simulink model "Modelo2R2021a"  (R2021a)
settings: Solver=VariableStepAuto  StartTime=0.0  StopTime=7e4  FixedStep=1  MaxStep=1  RelTol=1e-3
PostLoadFcn:
  | load('input_modelo_bateria.mat')
undefined symbols (not defined in the file or in its folder): alfa, beta, Cn, rest_time, SOC_MAX, SOC_MIN, Temperature, voc_fit
libraries: fl_lib x8, nesl_utility x7, ee_lib x2, simulink x1
settings Model: PacingRate=1000  Creator=eduardo.guimaraes  LastModifiedBy=mateu
settings SolverCC: AlgebraicLoopSolver=TrustRegion
settings DataIOCC: ReturnWorkspaceOutputs=off
settings DebuggingCC: SFMachineParentedDataDiag=warning  ArithmeticOperatorsInVariantConditions=warning
settings SFSimCC: CustomCodeUndefinedFunction=UseInterfaceOnly

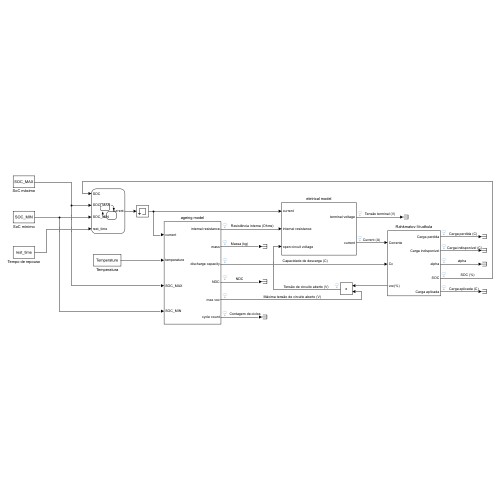
[thumbnail: Simulink's stored preview of the top-level diagram]
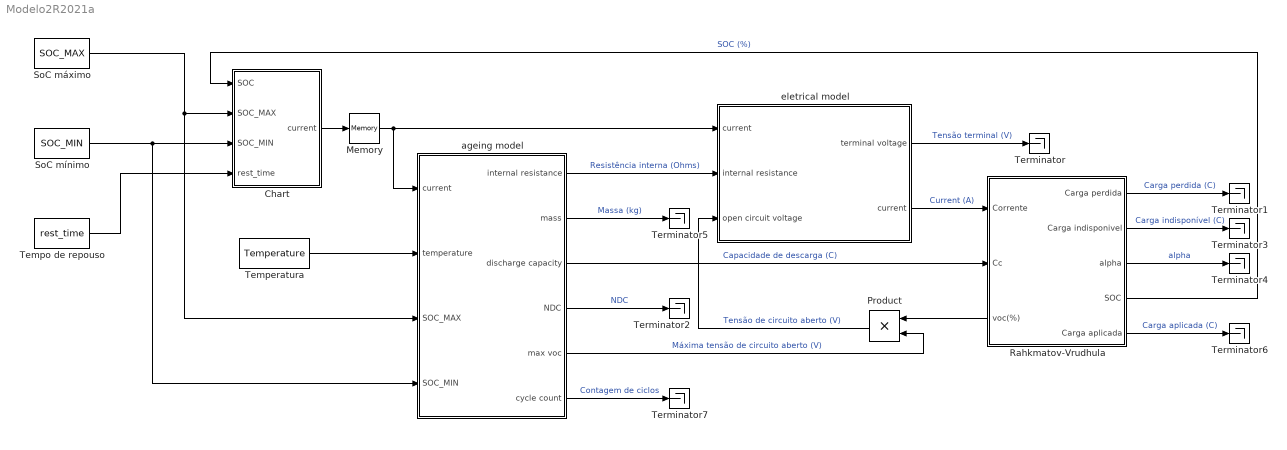
== system Modelo2R2021a ==
  Chart : Stateflow chart  TreatAsAtomicUnit=on
      settings: PortSchema="{\"entries\":[{\"content\":{\"sides\":[{\"content\":{\"connectorIds\":[\"In2\",\"In3\",\"In4\",\"In1\"]},\"type\":\"ConnectorPlacement.EquallySpacedRectSide\",\"uuid\":\"b79e6304-446b-4da0-b841-6a7e0125cfd5\"},{\"content\":{\"connectorIds\":[\"Out1\"],\"side\":\"RIGHT\"},\"type\":\"ConnectorPlacement.EquallySpacedRectSide\",\"uuid\":\"907ab61a-1d0a-45c7-8983-f54ad408e9d5\"},{\"content\":{\"connectorIds\":[],\"side\":\"TOP\"},\"type\":\"ConnectorPlacement.EquallySpacedRectSide\",\"uuid\":\"544cfd83-6b45-4625-b149-12de8a160085\"}]},\"type\":\"ConnectorPlacement.EquallySpacedConnector\",\"uuid\":\"2fa71fdc-98f6-47db-8b29-348eadeade42\"}],\"packageUris\":[\"http://schema.mathworks.com/mf0/Connector/R2020b\"],\"version\":\"1.0\"}"
  Memory : Memory
  Product : Product
  Rahkmatov-Vrudhula : Subsystem
      settings: PortSchema="{\"entries\":[{\"content\":{\"sides\":[{\"content\":{\"connectorIds\":[\"In1\",\"In2\",\"Out6\"]},\"type\":\"ConnectorPlacement.EquallySpacedRectSide\",\"uuid\":\"83f3e873-db9f-47d1-b7c3-7eda48a10b32\"},{\"content\":{\"connectorIds\":[\"Out1\",\"Out2\",\"Out3\",\"Out4\",\"Out5\"],\"side\":\"RIGHT\"},\"type\":\"ConnectorPlacement.EquallySpacedRectSide\",\"uuid\":\"48ac6012-cdb4-4752-bc48-afa50bea9f0a\"},{\"content\":{\"connectorIds\":[],\"side\":\"TOP\"},\"type\":\"ConnectorPlacement.EquallySpacedRectSide\",\"uuid\":\"9cdc78bf-a718-48f1-92e6-e4070151caee\"}]},\"type\":\"ConnectorPlacement.EquallySpacedConnector\",\"uuid\":\"a231f58d-8e16-4cb4-bc80-61541bcf90eb\"}],\"packageUris\":[\"http://schema.mathworks.com/mf0/Connector/R2020b\"],\"version\":\"1.0\"}"
  SoC máximo : Constant  Value=SOC_MAX
  SoC mínimo : Constant  Value=SOC_MIN
  Temperatura : Constant  Value=Temperature
  Tempo de repouso : Constant  Value=rest_time
  Terminator{,1..7} (8 alike) : Terminator
  ageing model : Subsystem
  eletrical model : Subsystem
  wires:
  Temperatura/1 -> ageing model/2(temperature)
  Rahkmatov-Vrudhula/4(SOC) -> Chart/2(SOC)  "SOC (%)"
  Tempo de repouso/1 -> Chart/1(rest_time)
  ageing model/3(discharge capacity) -> Rahkmatov-Vrudhula/2(Cc)  "Capacidade de descarga (C)"
  Chart/1(current) -> Memory/1
  Memory/1 -> eletrical model/1("current "), ageing model/1(current)
  SoC máximo/1 -> ageing model/3(SOC_MAX), Chart/3(SOC_MAX)
  SoC mínimo/1 -> ageing model/4(SOC_MIN), Chart/4(SOC_MIN)
  eletrical model/2(current) -> Rahkmatov-Vrudhula/1(Corrente)  "Current (A)"
  ageing model/1(internal resistance) -> eletrical model/2(internal resistance)  "Resistência interna (Ohms)"
  Rahkmatov-Vrudhula/6(voc(%)) -> Product/1
  ageing model/5(max voc) -> Product/2  "Máxima tensão de circuito aberto (V)"
  Product/1 -> eletrical model/3(open circuit voltage)  "Tensão de circuito aberto (V)"
  eletrical model/1(terminal voltage) -> Terminator/1  "Tensão terminal (V)"
  Rahkmatov-Vrudhula/1(Carga perdida) -> Terminator1/1  "Carga perdida (C)"
  Rahkmatov-Vrudhula/2(Carga indisponivel) -> Terminator3/1  "Carga indisponível (C)"
  Rahkmatov-Vrudhula/3(alpha) -> Terminator4/1  "alpha"
  ageing model/4(NDC) -> Terminator2/1  "NDC"
  ageing model/2(mass) -> Terminator5/1  "Massa (kg)"
  Rahkmatov-Vrudhula/5(Carga aplicada) -> Terminator6/1  "Carga aplicada (C)"
  ageing model/6(cycle count) -> Terminator7/1  "Contagem de ciclos"

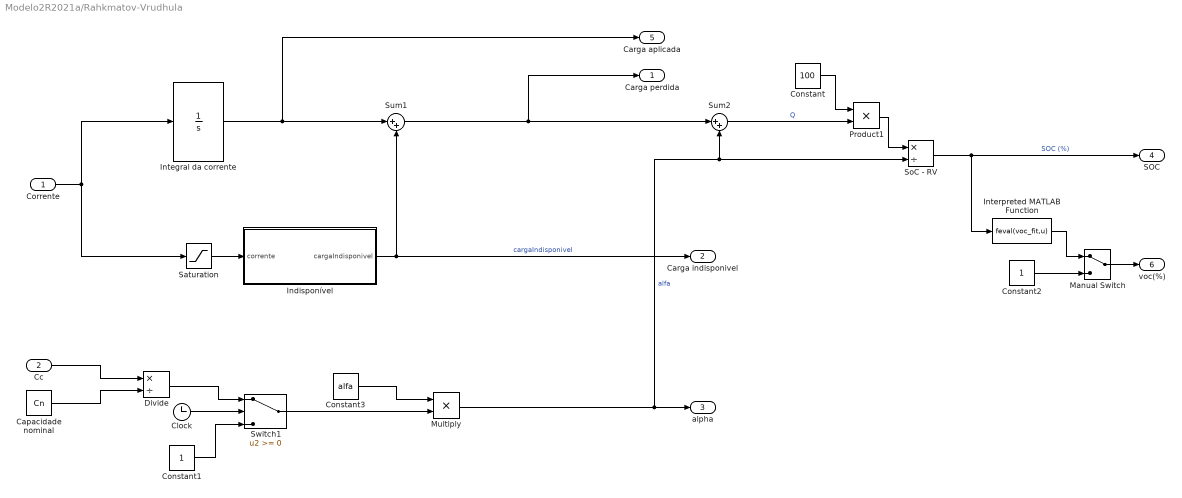
== system Modelo2R2021a/Rahkmatov-Vrudhula ==
  Corrente : Inport
  Cc : Inport  Port=2
  Capacidade nominal : Constant  Value=Cn
  Clock : Clock
  Constant : Constant  Value=100
  Constant1 : Constant
  Constant2 : Constant
  Constant3 : Constant  Value=alfa
  Divide : Product  Inputs=*/
  Indisponível : Subsystem
  Integral da corrente : Integrator  LimitOutput=on  UpperSaturationLimit=0  LowerSaturationLimit=-alfa
  Interpreted MATLAB Function : MATLABFcn  MATLABFcn=feval(voc_fit,u)
  Manual Switch : ManualSwitch
  Multiply : Product
  Product1 : Product
  Saturation : Saturate  UpperLimit=0  LowerLimit=-Inf
  SoC - RV : Product  Inputs=*/
  Sum1 : Sum  Inputs=|++
  Sum2 : Sum  Inputs=|++
  Switch1 : Switch
  Carga perdida : Outport  VectorParamsAs1DForOutWhenUnconnected=off
  Carga indisponivel : Outport  Port=2  VectorParamsAs1DForOutWhenUnconnected=off
  alpha : Outport  Port=3  VectorParamsAs1DForOutWhenUnconnected=off
  SOC : Outport  Port=4
  Carga aplicada : Outport  Port=5  VectorParamsAs1DForOutWhenUnconnected=off
  voc(%) : Outport  Port=6
  wires:
  Indisponível/1(cargaIndisponivel) -> Sum1/2, Carga indisponivel/1  "cargaIndisponivel"
  Switch1/1 -> Multiply/2
  Constant3/1 -> Multiply/1
  Constant/1 -> Product1/1
  Multiply/1 -> Sum2/2, SoC - RV/2, alpha/1  "alfa"
  Product1/1 -> SoC - RV/1
  SoC - RV/1 -> Interpreted MATLAB Function/1, SOC/1  "SOC (%)"
  Saturation/1 -> Indisponível/1(corrente)
  Sum2/1 -> Product1/2  "Q"
  Constant1/1 -> Switch1/3
  Clock/1 -> Switch1/2
  Divide/1 -> Switch1/1
  Cc/1 -> Divide/1
  Capacidade nominal/1 -> Divide/2
  Integral da corrente/1 -> Carga aplicada/1, Sum1/1
  Corrente/1 -> Integral da corrente/1, Saturation/1
  Sum1/1 -> Carga perdida/1, Sum2/1
  Manual Switch/1 -> voc(%)/1
  Interpreted MATLAB Function/1 -> Manual Switch/1
  Constant2/1 -> Manual Switch/2

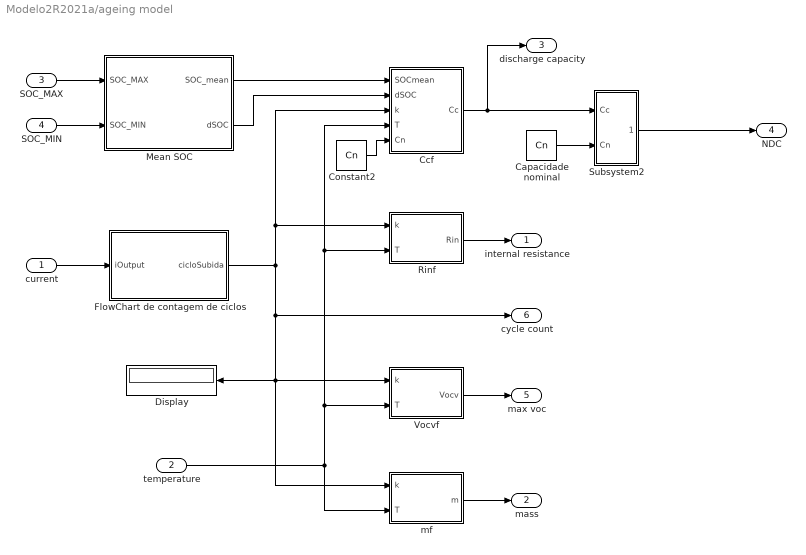
== system Modelo2R2021a/ageing model ==
  current : Inport
  temperature : Inport  Port=2
  SOC_MAX : Inport  Port=3
  SOC_MIN : Inport  Port=4
  Capacidade nominal : Constant  Value=Cn
  Ccf : MATLAB Function  TreatAsAtomicUnit=on
  Constant2 : Constant  Value=Cn
  Display : Display
  FlowChart de contagem de ciclos : Stateflow chart  TreatAsAtomicUnit=on
  Mean SOC : Subsystem
  Rinf : MATLAB Function  TreatAsAtomicUnit=on
  Subsystem2 : Subsystem
  Vocvf : MATLAB Function  TreatAsAtomicUnit=on
  mf : MATLAB Function  TreatAsAtomicUnit=on
  internal resistance : Outport
  mass : Outport  Port=2
  discharge capacity : Outport  Port=3
  NDC : Outport  Port=4
  max voc : Outport  Port=5
  cycle count : Outport  Port=6
  wires:
  Vocvf/1(Vocv) -> max voc/1
  temperature/1 -> mf/2(T), Vocvf/2(T), Rinf/2(T), Ccf/4(T)
  Rinf/1(Rin) -> internal resistance/1
  mf/1(m) -> mass/1
  current/1 -> FlowChart de contagem de ciclos/1(iOutput)
  Ccf/1(Cc) -> discharge capacity/1, Subsystem2/1(Cc)
  Subsystem2/1(NDC) -> NDC/1
  Capacidade nominal/1 -> Subsystem2/2(Cn)
  Constant2/1 -> Ccf/5(Cn)
  SOC_MAX/1 -> Mean SOC/1(SOC_MAX)
  SOC_MIN/1 -> Mean SOC/2(SOC_MIN)
  Mean SOC/1(SOC_mean) -> Ccf/1(SOCmean)
  Mean SOC/2(dSOC) -> Ccf/2(dSOC)
  FlowChart de contagem de ciclos/1(cicloSubida) -> Ccf/3(k), Rinf/1(k), cycle count/1, Display/1, mf/1(k), Vocvf/1(k)

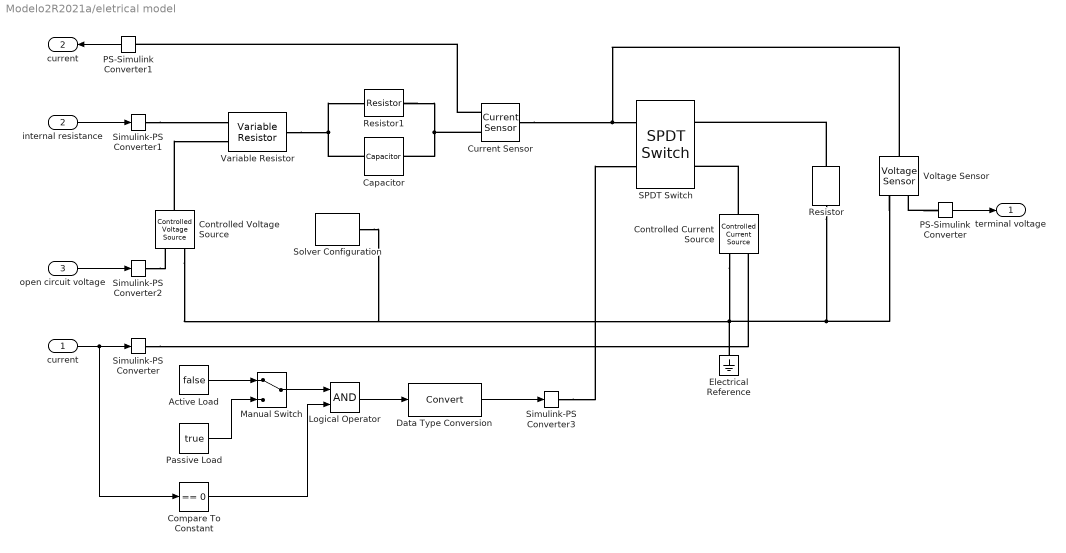
== system Modelo2R2021a/eletrical model ==
  "current " : Inport
  internal resistance : Inport  Port=2
  open circuit voltage : Inport  Port=3
  Active Load : Constant  Value=false
  Capacitor : fl_lib/Electrical/Electrical Elements/Capacitor  c=500 F  r=1e-6 Ohm  g=0 1/Ohm  i_specify=off  i_priority=None  i=0 A  i_nominal_specify=off  i_nominal_unit=A  i_nominal_value=1  v_specify=off  v_priority=None  v=0 V  v_nominal_specify=off  v_nominal_unit=V  v_nominal_value=1  vc_specify=off  vc_priority=High  vc=0 V  vc_nominal_specify=off  vc_nominal_unit=V  vc_nominal_value=1
      settings: SourceProductBaseCode=PW,SS,VE
  Compare To Constant : simulink/Logic and Bit Operations/Compare To Constant  relop===  const=0  OutDataTypeStr=boolean
  Controlled Current Source : fl_lib/Electrical/Electrical Sources/Controlled Current Source
      settings: SourceProductBaseCode=PW,SS,VE
  Controlled Voltage Source : fl_lib/Electrical/Electrical Sources/Controlled Voltage Source
      settings: SourceProductBaseCode=PW,SS,VE
  Current Sensor : fl_lib/Electrical/Electrical Sensors/Current Sensor
      settings: SourceProductBaseCode=PW,SS,VE
  Data Type Conversion : DataTypeConversion
  Electrical Reference : fl_lib/Electrical/Electrical Elements/Electrical Reference
      settings: SourceProductBaseCode=PW,SS,VE
  Logical Operator : Logic  AllPortsSameDT=off  OutDataTypeStr=boolean
  Manual Switch : ManualSwitch
  PS-Simulink Converter : nesl_utility/PS-Simulink Converter  PhysicalDomain=network_engine_domain  SubClassName=ps_output  LeftPortType=input  RightPortType=output  PseudoPeriodic=off  Frequencies=[]  VectorFormat=inherit  Unit=inherit  AffineConversion=off
      settings: SourceProductBaseCode=SS,PW,VE
  PS-Simulink Converter1 : nesl_utility/PS-Simulink Converter  PhysicalDomain=network_engine_domain  SubClassName=ps_output  LeftPortType=input  RightPortType=output  PseudoPeriodic=off  Frequencies=[]  VectorFormat=inherit  Unit=inherit  AffineConversion=off
      settings: SourceProductBaseCode=SS,PW,VE
  Passive Load : Constant  Value=true
  Resistor : ee_lib/Passive/Resistor  R=0.1 Ohm  enable_R_tol=0  R_tol=5  tol_distribution=1  nSigma=4  enable_operating_limits=0  operating_limit_action=2  max_working_voltage=100 V  power_rating=1 W  enable_faults=0  fault_action=1  R_faulted=inf Ohm  enable_temporal_fault=0  t_fault=1 s  enable_behavioral_fault=0  max_permissible_current=1 A  t_fail_on_current=1 s  noise_mode=0  sample_time=1e-3 s  repeatability=1  auto_seed=3499211588  user_seed=0  Tdevice=25 degC  power_derating_T1=70 degC  power_derating_T2=155 degC  operating_temperature_range_vec=[-50, 150] degC  alpha=3.93e-3 1/K  Tmeas=25 degC  thermal_mass=100 J/K  temperature_specify=off  temperature_priority=High  temperature=298.15 K  temperature_nominal_specify=off  temperature_nominal_unit=K  temperature_nominal_value=1
  Resistor1 : fl_lib/Electrical/Electrical Elements/Resistor  R=1e-6 Ohm  i_specify=off  i_priority=None  i=0 A  i_nominal_specify=off  i_nominal_unit=A  i_nominal_value=1  v_specify=off  v_priority=None  v=0 V  v_nominal_specify=off  v_nominal_unit=V  v_nominal_value=1
      settings: SourceProductBaseCode=PW,SS,VE
  SPDT Switch : ee_lib/Switches & Breakers/SPDT Switch  R_closed=0.01 Ohm  G_open=1e-6 S  Threshold=0.5 V  Width=0 V  model_dynamics=0  t_on=1e-3 s  t_off=1e-3 s  initial_vT=0 V
      settings: SourceProductBaseCode=PS
  Simulink-PS Converter : nesl_utility/Simulink-PS Converter  PhysicalDomain=network_engine_domain  SubClassName=ps_input  LeftPortType=input  RightPortType=output  PseudoPeriodic=off  Frequencies=[]  NoiseDistribution=none  NoiseParameters=[]  Unit=1  AffineConversion=off  FilteringAndDerivatives=zero  SimscapeFilterOrder=1  InputFilterTimeConstant=0.001  UdotUserProvided=0
      settings: SourceProductBaseCode=SS,PW,VE
  Simulink-PS Converter1 : nesl_utility/Simulink-PS Converter  PhysicalDomain=network_engine_domain  SubClassName=ps_input  LeftPortType=input  RightPortType=output  PseudoPeriodic=off  Frequencies=[]  NoiseDistribution=none  NoiseParameters=[]  Unit=1  AffineConversion=off  FilteringAndDerivatives=zero  SimscapeFilterOrder=1  InputFilterTimeConstant=0.001  UdotUserProvided=0
      settings: SourceProductBaseCode=SS,PW,VE
  Simulink-PS Converter2 : nesl_utility/Simulink-PS Converter  PhysicalDomain=network_engine_domain  SubClassName=ps_input  LeftPortType=input  RightPortType=output  PseudoPeriodic=off  Frequencies=[]  NoiseDistribution=none  NoiseParameters=[]  Unit=1  AffineConversion=off  FilteringAndDerivatives=zero  SimscapeFilterOrder=1  InputFilterTimeConstant=0.001  UdotUserProvided=0
      settings: SourceProductBaseCode=SS,PW,VE
  Simulink-PS Converter3 : nesl_utility/Simulink-PS Converter  PhysicalDomain=network_engine_domain  SubClassName=ps_input  LeftPortType=input  RightPortType=output  PseudoPeriodic=off  Frequencies=[]  NoiseDistribution=none  NoiseParameters=[]  Unit=1  AffineConversion=off  FilteringAndDerivatives=provide  SimscapeFilterOrder=1  InputFilterTimeConstant=0.001  UdotUserProvided=0
      settings: SourceProductBaseCode=SS,PW,VE
  Solver Configuration : nesl_utility/Solver Configuration  PhysicalDomain=network_engine_domain  SubClassName=solver  LeftPortType=input  RightPortType=generic  Tones=[]  Harmonics=[]  SimulateNoise=off  Profile=off  UseLocalSampling=off  EnableSwitchedLinearOptims=on  FrequencyDomain=off  UseCCode=off  RelTol=0.001  AbsTol=0.001  MinStep=1e-09  ToWorkspace=off  RevertToSquareIcSolve=off  NumHomotopyIterations=100  PhasorMode=off  PhasorModeNumHarmonics=1  IndexReductionMethod=DerivativeReplacement  DoDC=off  ResidualTolerance=1e-09  UseLocalSolver=off  LocalSolverChoice=NE_BACKWARD_EULER_ADVANCER  LocalSolverSampleTime=0.001  DoFixedCost=off  MaxNonlinIter=3  MaxModeIter=2  ComputeImpulses=off  ImpulseIterations=2  LinearAlgebra=auto  LinearAlgebraNumThread=0  EquationFormulation=NE_TIME_EF  DelaysMemoryBudget=1024  AutomaticFiltering=on  FilteringTimeConstant=0.001  PartitionStorageMethod=AS_NEEDED  PartitionMemoryBudget=1024  PartitionMethod=ROBUST
      settings: SourceProductBaseCode=SS,PW,VE
  Variable Resistor : fl_lib/Electrical/Electrical Elements/Variable Resistor  Rmin=0 Ohm  i_specify=off  i_priority=None  i=0 A  i_nominal_specify=off  i_nominal_unit=A  i_nominal_value=1  v_specify=off  v_priority=None  v=0 V  v_nominal_specify=off  v_nominal_unit=V  v_nominal_value=1
      settings: SourceProductBaseCode=PW,SS,VE
  Voltage Sensor : fl_lib/Electrical/Electrical Sensors/Voltage Sensor
      settings: SourceProductBaseCode=PW,SS,VE
  terminal voltage : Outport
  current : Outport  Port=2
  wires:
  open circuit voltage/1 -> Simulink-PS Converter2/1
  "current "/1 -> Compare To Constant/1, Simulink-PS Converter/1
  PS-Simulink Converter1/1 -> current/1
  internal resistance/1 -> Simulink-PS Converter1/1
  PS-Simulink Converter/1 -> terminal voltage/1
  Compare To Constant/1 -> Logical Operator/2
  Logical Operator/1 -> Data Type Conversion/1
  Data Type Conversion/1 -> Simulink-PS Converter3/1
  Active Load/1 -> Manual Switch/1
  Passive Load/1 -> Manual Switch/2
  Manual Switch/1 -> Logical Operator/1
  connections:
  Variable Resistor/RConn1 -- Capacitor/LConn1 -- Resistor1/LConn1
  Voltage Sensor/RConn2 -- Controlled Voltage Source/RConn2 -- Solver Configuration/RConn1 -- Controlled Current Source/RConn2 -- Electrical Reference/LConn1 -- Resistor/RConn1
  Controlled Voltage Source/LConn1 -- Variable Resistor/LConn2
  Simulink-PS Converter/RConn1 -- Controlled Current Source/RConn1
  PS-Simulink Converter/LConn1 -- Voltage Sensor/RConn1
  Simulink-PS Converter1/RConn1 -- Variable Resistor/LConn1
  Simulink-PS Converter2/RConn1 -- Controlled Voltage Source/RConn1
  Resistor1/RConn1 -- Current Sensor/RConn2 -- Capacitor/RConn1
  Voltage Sensor/LConn1 -- Current Sensor/LConn1 -- SPDT Switch/LConn2
  Current Sensor/RConn1 -- PS-Simulink Converter1/LConn1
  Controlled Current Source/LConn1 -- SPDT Switch/RConn1
  Resistor/LConn1 -- SPDT Switch/RConn2
  Simulink-PS Converter3/RConn1 -- SPDT Switch/LConn1

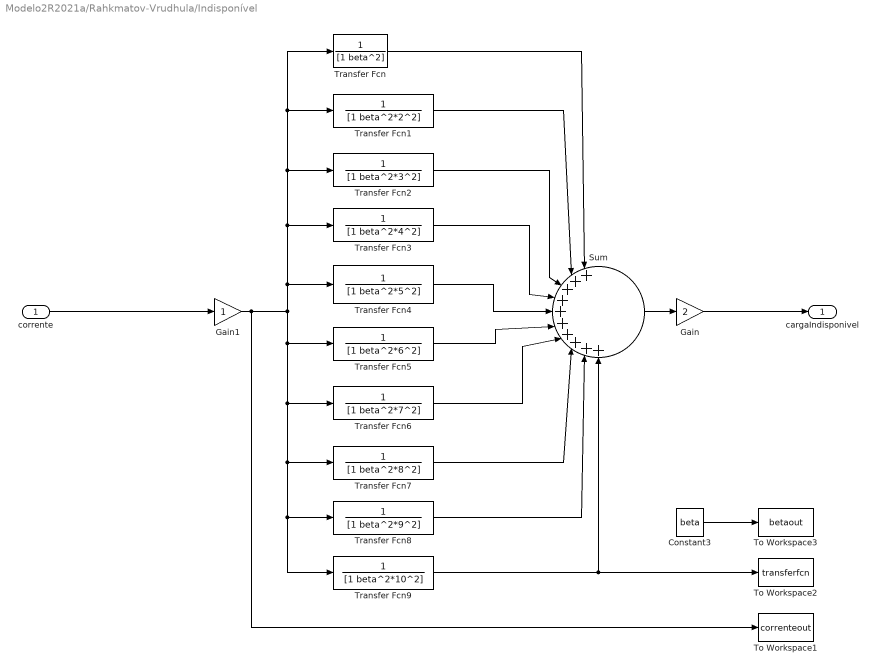
== system Modelo2R2021a/Rahkmatov-Vrudhula/Indisponível ==
  corrente : Inport
  Constant3 : Constant  Value=beta
  Gain : Gain  Gain=2
  Gain1 : Gain
  Sum : Sum  Inputs=|++++++++++
  To Workspace1 : ToWorkspace  VariableName=correnteout  SampleTime=-1
      settings: Save2DSignal=2-D array (concatenate along first dimension)
  To Workspace2 : ToWorkspace  VariableName=transferfcn  SampleTime=-1
      settings: Save2DSignal=2-D array (concatenate along first dimension)
  To Workspace3 : ToWorkspace  VariableName=betaout  SampleTime=-1
      settings: Save2DSignal=2-D array (concatenate along first dimension)
  Transfer Fcn : TransferFcn  Denominator=[1 beta^2]
  Transfer Fcn1 : TransferFcn  Denominator=[1 beta^2*2^2]
  Transfer Fcn2 : TransferFcn  Denominator=[1 beta^2*3^2]
  Transfer Fcn3 : TransferFcn  Denominator=[1 beta^2*4^2]
  Transfer Fcn4 : TransferFcn  Denominator=[1 beta^2*5^2]
  Transfer Fcn5 : TransferFcn  Denominator=[1 beta^2*6^2]
  Transfer Fcn6 : TransferFcn  Denominator=[1 beta^2*7^2]
  Transfer Fcn7 : TransferFcn  Denominator=[1 beta^2*8^2]
  Transfer Fcn8 : TransferFcn  Denominator=[1 beta^2*9^2]
  Transfer Fcn9 : TransferFcn  Denominator=[1 beta^2*10^2]
  cargaIndisponivel : Outport  VectorParamsAs1DForOutWhenUnconnected=off
  wires:
  Transfer Fcn/1 -> Sum/1
  Transfer Fcn1/1 -> Sum/2
  Transfer Fcn2/1 -> Sum/3
  Transfer Fcn3/1 -> Sum/4
  Transfer Fcn4/1 -> Sum/5
  Transfer Fcn5/1 -> Sum/6
  Transfer Fcn6/1 -> Sum/7
  Transfer Fcn7/1 -> Sum/8
  Transfer Fcn8/1 -> Sum/9
  Transfer Fcn9/1 -> To Workspace2/1, Sum/10
  Sum/1 -> Gain/1
  Gain1/1 -> To Workspace1/1, Transfer Fcn5/1, Transfer Fcn6/1, Transfer Fcn7/1, Transfer Fcn8/1, Transfer Fcn9/1, Transfer Fcn4/1, Transfer Fcn3/1, Transfer Fcn2/1, Transfer Fcn1/1, Transfer Fcn/1
  corrente/1 -> Gain1/1
  Gain/1 -> cargaIndisponivel/1
  Constant3/1 -> To Workspace3/1

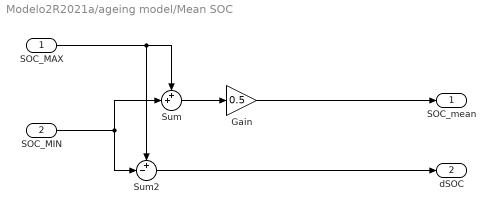
== system Modelo2R2021a/ageing model/Mean SOC ==
  SOC_MAX : Inport
  SOC_MIN : Inport  Port=2
  Gain : Gain  Gain=0.5
  Sum : Sum  Inputs=++|
  Sum2 : Sum  Inputs=+-|
  SOC_mean : Outport
  dSOC : Outport  Port=2
  wires:
  Sum/1 -> Gain/1
  SOC_MIN/1 -> Sum/2, Sum2/2
  SOC_MAX/1 -> Sum/1, Sum2/1
  Sum2/1 -> dSOC/1
  Gain/1 -> SOC_mean/1

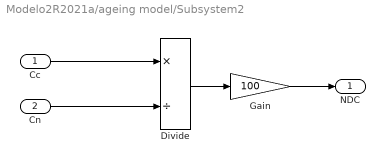
== system Modelo2R2021a/ageing model/Subsystem2 ==
  Cc : Inport
  Cn : Inport  Port=2
  Divide : Product  Inputs=*/
  Gain : Gain  Gain=100
  NDC : Outport
  wires:
  Divide/1 -> Gain/1
  Cn/1 -> Divide/2
  Gain/1 -> NDC/1
  Cc/1 -> Divide/1

== matlab function Modelo2R2021a/ageing model/Rinf ==
  data: k input; Rin output; T input
function Rin = fcn(k,T)

       x = (k-9000)/6326;
       y = (T-31.67)/10.57;
       
%        where x is normalized by mean 9000 and std 6326
%        and where y is normalized by mean 31.67 and std 10.57
% Coefficients (with 95% confidence bounds):
       p00 =    0.003956;%  (0.003728, 0.004184)
       p10 =   0.0006753;%  (0.0004339, 0.0009166)
       p01 =  -1.804e-05;%  (-0.0001419, 0.0001059)
       p20 =   0.0005921;%  (0.000144, 0.00104)
       p11 =   0.0002673;%  (4.651e-05, 0.0004881)
       p02 =   3.119e-05;%  (-0.0001491, 0.0002115)
       p30 =   0.0001137;%  (-7.891e-06, 0.0002354)
       p21 =   0.0002022;%  (0.0001025, 0.0003019)
       p12 =  -0.0002286;%  (-0.0003492, -0.0001081)
       p40 =  -1.788e-05;%  (-0.0002076, 0.0001718)
       p31 =  -1.552e-05;%  (-0.0001407, 0.0001096)
       p22 =  -0.0001674;%  (-0.0003125, -2.232e-05)

       %Linear model Poly42:
     Rin = p00 + p10*x + p01*y + p20*x^2 + p11*x*y + p02*y^2 + p30*x^3 + p21*x^2*y ...
                    + p12*x*y^2 + p40*x^4 + p31*x^3*y + p22*x^2*y^2;

       
% Goodness of fit:
%   SSE: 9.784e-08
%   R-square: 0.991
%   Adjusted R-square: 0.9746
%   RMSE: 0.0001277

== matlab function Modelo2R2021a/ageing model/Ccf ==
  data: SOCmean input; dSOC input; k input; Cc output; T input; Cn input
function Cc = fcn(SOCmean, dSOC,k,T,Cn)
% Coeficients model Saxena2016
        k1 = 3.25;
        k2 = 3.25;
        k3 = -2.25;
% Coefficients (with 95% confidence bounds):
       p00 =       56.02;%  (53.93, 58.1)
       p10 =      -10.53;%  (-13.71, -7.36)
       p01 =       0.869;%  (-0.7052, 2.443)
       p20 =      -4.808;%  (-6.007, -3.609)
       p11 =      -1.445;%  (-2.534, -0.3554)
       p02 =      -1.223;%  (-2.763, 0.3179)
       p30 =      -2.931;%  (-4.53, -1.332)
       p21 =       -1.55;%  (-2.783, -0.3163)
       p12 =    -0.09181;%  (-1.677, 1.493)

       x = (k-9000)/6326;
       y = (T-31.67)/10.57;
       
%Linear model Poly32:
     fcn = p00 + p10*x + p01*y + p20*x^2 + p11*x*y + p02*y^2 + p30*x^3 + p21*x^2*y + p12*x*y^2;

     Cc = (100 - k1*SOCmean/100*(1+k2*dSOC/100+k3*(dSOC/100)^2) )/100*fcn
                    
%       where x is normalized by mean 9000 and std 6326
%       and where y is normalized by mean 31.67 and std 10.57


% Goodness of fit:
%   SSE: 29.68
%   R-square: 0.9934
%   Adjusted R-square: 0.9875
%   RMSE: 1.816

== stateflow chart Modelo2R2021a/ageing model/FlowChart de contagem de ciclos ==
  note: Automato de contagem de ciclos
  state Respouso
  state Descarregando
  state Carregando
  (default) -> Respouso
  Respouso -> Descarregando [order 1] : [iOutput<0]
  Descarregando -> Respouso [order 1] : [iOutput==0]
  Respouso -> Carregando [order 2] : [iOutput>0]{cicloSubida = cicloSubida + 1}
  Carregando -> Respouso [order 2] : [iOutput==0]
  Carregando -> Descarregando [order 1] : [iOutput<0]
  Descarregando -> Carregando [order 2] : [iOutput>0]{cicloSubida = cicloSubida + 1}
  data: cicloSubida output =0; iOutput input

== matlab function Modelo2R2021a/ageing model/Vocvf ==
  data: k input; Vocv output; T input
function Vocv = fcn(k,T)

%Coefficients (with 95% confidence bounds):
       p00 =       12.46;%  (12.4, 12.53)
       p10 =      0.2911;%  (0.2589, 0.3233)
       p01 =     0.03352;%  (-0.0006909, 0.06772)
       p20 =      0.0383;%  (-0.0004375, 0.07703)
       p11 =     0.02935;%  (-0.003774, 0.06248)
       p02 =    -0.01441;%  (-0.06418, 0.03537)

       x = (k-9000)/6326;
       y = (T-31.67)/10.57;
       
%Linear model Poly22:
     Vocv = p00 + p10*x + p01*y + p20*x^2 + p11*x*y + p02*y^2;
%       where x is normalized by mean 9000 and std 6326
%       and where y is normalized by mean 31.67 and std 10.57

%Goodness of fit:
%  SSE: 0.04454
%  R-square: 0.971
%  Adjusted R-square: 0.9588
%  RMSE: 0.06092

== matlab function Modelo2R2021a/ageing model/mf ==
  data: k input; m output; T input
function m = fcn(k,T)

%Coefficients (with 95% confidence bounds):
       p00 =       19.64;%  (19.58, 19.69)
       p10 =     -0.5246;%  (-0.606, -0.4431)
       p01 =    -0.08727;%  (-0.1277, -0.04686)
       p20 =        0.06;%  (0.02923, 0.09077)
       p11 =    -0.04133;%  (-0.0693, -0.01337)
       p02 =    -0.04346;%  (-0.08301, -0.003916)
       p30 =     0.02928;%  (-0.01177, 0.07033)
       p21 =    -0.02198;%  (-0.05365, 0.009682)
       p12 =      0.0413;%  (0.0006076, 0.082)

       x = (k-9000)/6326;
       y = (T-31.67)/10.57;
       
% Linear model Poly32:
     m = p00 + p10*x + p01*y + p20*x^2 + p11*x*y + p02*y^2 + p30*x^3 + p21*x^2*y ...
                    + p12*x*y^2;
%        where x is normalized by mean 9000 and std 6326
%        and where y is normalized by mean 31.67 and std 10.57


% Goodness of fit:
%   SSE: 0.01956
%   R-square: 0.9946
%   Adjusted R-square: 0.9898
%   RMSE: 0.04662

== stateflow chart Modelo2R2021a/Chart ==
  settings: executeAtInitialization=1
  state Descarga
    current=-40;
  state Repouso
    current=0;
  state Recarga
    current=60;
  (junction 23) -> Descarga [order 1] : [SOC>=SOC_MAX]
  Descarga -> Recarga : [SOC<=SOC_MIN]
  (default) -> Repouso
  Repouso -> (junction 23) : [after(rest_time,sec)]
  (junction 23) -> Recarga [order 2]
  Recarga -> Repouso : [SOC>=SOC_MAX]
  data: rest_time input; current output; SOC input; SOC_MAX input; SOC_MIN input
